simulink model "2pointDFT"  (R2021b)
settings: Solver=VariableStepAuto  StartTime=0.0  StopTime=10.0  RelTol=1e-3
settings Model: Creator=Admin  LastModifiedBy=Admin

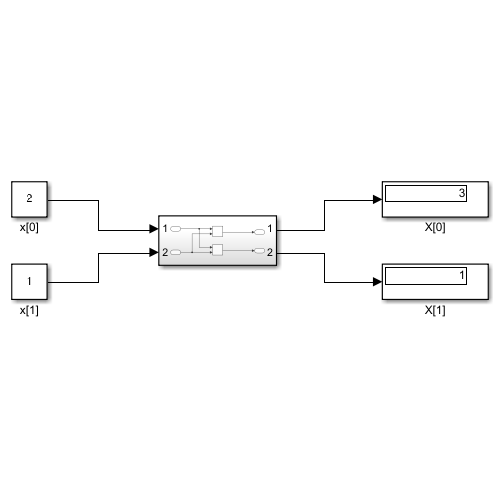
[thumbnail: Simulink's stored preview of the top-level diagram]
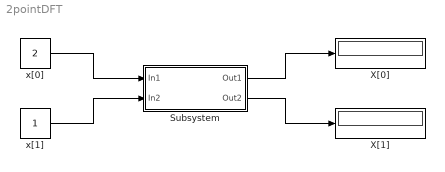
== system 2pointDFT ==
  Subsystem : Subsystem
  X[0] : Display
  X[1] : Display
  x[0] : Constant  Value=2
  x[1] : Constant
  wires:
  x[0]/1 -> Subsystem/1(In1)
  Subsystem/1(Out1) -> X[0]/1
  x[1]/1 -> Subsystem/2(In2)
  Subsystem/2(Out2) -> X[1]/1

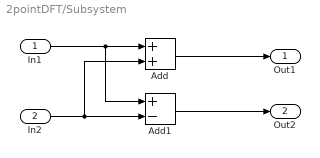
== system 2pointDFT/Subsystem ==
  In1 : Inport
  In2 : Inport  Port=2
  Add : Sum
  Add1 : Sum  Inputs=+-
  Out1 : Outport
  Out2 : Outport  Port=2
  wires:
  In1/1 -> Add1/1, Add/1
  In2/1 -> Add/2, Add1/2
  Add/1 -> Out1/1
  Add1/1 -> Out2/1
